simulink model "PerturbedMeanOrbitPropagator"  (R2023a)
settings: Solver=ode4  StartTime=0.0  StopTime=10.0  FixedStep=dt  MaxStep=max_step_size  RelTol=relative_tolerance
undefined symbols (not defined in the file or in its folder): J2_flag, srp_flag
settings Model: Creator=ndelurgio  LastModifiedBy=ndelurgio

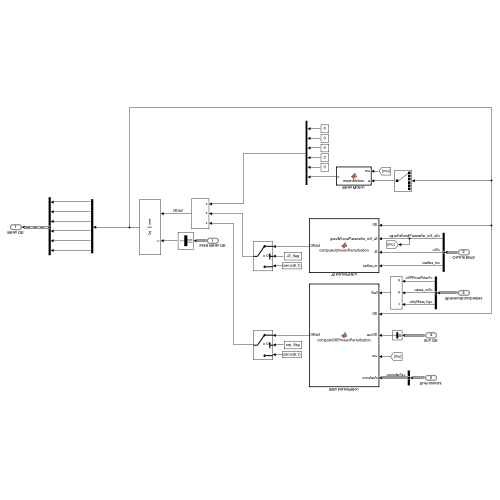
[thumbnail: Simulink's stored preview of the top-level diagram]
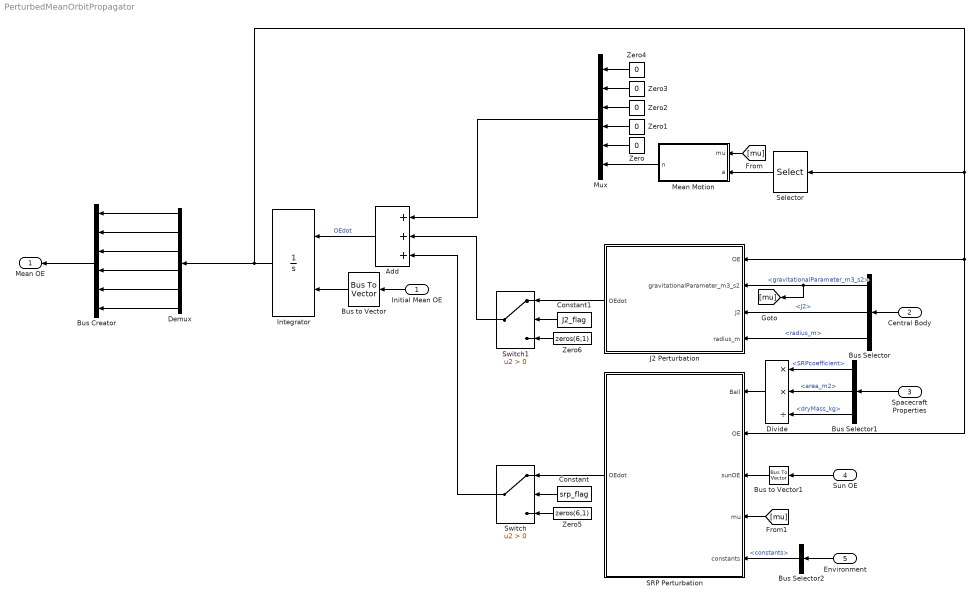
== system PerturbedMeanOrbitPropagator ==
  Initial Mean OE : Inport  OutDataTypeStr=Bus: meanOrbitElements
  Central Body : Inport  Port=2  OutDataTypeStr=Bus: planetProperties
  Spacecraft Properties : Inport  Port=3  OutDataTypeStr=Bus: properties
  Sun OE : Inport  Port=4  OutDataTypeStr=Bus: osculatingOrbitElements
  Environment : Inport  Port=5  OutDataTypeStr=Bus: environmentBus
  Add : Sum  Inputs=+++
  Bus Creator : BusCreator  Inputs=6  OutDataTypeStr=Bus: meanOrbitElements  NonVirtualBus=on
      settings: InheritFromInputs=off
  Bus Selector : BusSelector  OutputSignals=gravitationalParameter_m3_s2,J2,radius_m
  Bus Selector1 : BusSelector  OutputSignals=SRPcoefficient,area_m2,dryMass_kg
  Bus Selector2 : BusSelector  OutputSignals=constants
  Bus to Vector : BusToVector
  Bus to Vector1 : BusToVector
  Constant : Constant  Value=srp_flag
  Constant1 : Constant  Value=J2_flag
  Demux : Demux  Outputs=6
  Divide : Product  Inputs=**/
  Integrator : Integrator  InitialConditionSource=external
  J2 Perturbation : MATLAB Function  TreatAsAtomicUnit=on
  Mean Motion : MATLAB Function  TreatAsAtomicUnit=on
  Mux : Mux  Inputs=6
  SRP Perturbation : MATLAB Function  TreatAsAtomicUnit=on
  Selector : Selector  InputPortWidth=6  IndexOptions=Index vector (dialog)  Indices=[1]  OutputSizes=1
  Switch : Switch  Criteria=u2 > Threshold  SaturateOnIntegerOverflow=off  InputSameDT=off
  Switch1 : Switch  Criteria=u2 > Threshold  SaturateOnIntegerOverflow=off  InputSameDT=off
  Zero{,1..4} (5 alike) : Constant  Value=0  OutDataTypeStr=Inherit: Inherit via back propagation
  Zero5 : Constant  Value=zeros(6,1)  OutDataTypeStr=Inherit: Inherit via back propagation
  Zero6 : Constant  Value=zeros(6,1)  OutDataTypeStr=Inherit: Inherit via back propagation
  Mean OE : Outport  OutDataTypeStr=Bus: meanOrbitElements
  wires:
  Initial Mean OE/1 -> Bus to Vector/1
  Bus to Vector/1 -> Integrator/2
  Add/1 -> Integrator/1  "OEdot"
  Mean Motion/1(n) -> Mux/6
  Zero/1 -> Mux/5
  Zero1/1 -> Mux/4
  Zero2/1 -> Mux/3
  Zero3/1 -> Mux/2
  Zero4/1 -> Mux/1
  Mux/1 -> Add/1
  Integrator/1 -> Demux/1, Selector/1, J2 Perturbation/1(OE), SRP Perturbation/2(OE)
  Selector/1 -> Mean Motion/2(a)
  Central Body/1 -> Bus Selector/1
  Bus Selector/2 -> J2 Perturbation/3(J2)  "<J2>"
  Bus Selector/1 -> [mu], J2 Perturbation/2(gravitationalParameter_m3_s2)  "<gravitationalParameter_m3_s2>"
  Bus Selector/3 -> J2 Perturbation/4(radius_m)  "<radius_m>"
  [mu] -> Mean Motion/1(mu)
  SRP Perturbation/1(OEdot) -> Switch/1
  [mu] -> SRP Perturbation/4(mu)
  Spacecraft Properties/1 -> Bus Selector1/1
  Sun OE/1 -> Bus to Vector1/1
  Bus to Vector1/1 -> SRP Perturbation/3(sunOE)
  Bus Selector1/1 -> Divide/1  "<SRPcoefficient>"
  Bus Selector1/2 -> Divide/2  "<area_m2>"
  Divide/1 -> SRP Perturbation/1(Ball)
  Bus Selector1/3 -> Divide/3  "<dryMass_kg>"
  Bus Selector2/1 -> SRP Perturbation/5(constants)  "<constants>"
  Environment/1 -> Bus Selector2/1
  Demux/1 -> Bus Creator/1
  Demux/2 -> Bus Creator/2
  Demux/3 -> Bus Creator/3
  Demux/4 -> Bus Creator/4
  Demux/5 -> Bus Creator/5
  Demux/6 -> Bus Creator/6
  Bus Creator/1 -> Mean OE/1
  Constant/1 -> Switch/2
  Zero5/1 -> Switch/3
  Switch/1 -> Add/3
  J2 Perturbation/1(OEdot) -> Switch1/1
  Zero6/1 -> Switch1/3
  Constant1/1 -> Switch1/2
  Switch1/1 -> Add/2

== matlab function PerturbedMeanOrbitPropagator/J2 Perturbation ==
  data: OE input; OEdot output; gravitationalParameter_m3_s2 input; J2 input; radius_m input
function OEdot = computeJ2meanPerturbation(OE,gravitationalParameter_m3_s2,J2,radius_m)
OEdot = computeJ2meanPerturbation(OE,gravitationalParameter_m3_s2,J2,radius_m);
end

== matlab function PerturbedMeanOrbitPropagator/Mean Motion ==
  data: mu input; n output; a input
function n = meanMotion (mu, a)
n = meanMotion (mu, a);
end

== matlab function PerturbedMeanOrbitPropagator/SRP Perturbation ==
  data: Ball input; OEdot output; OE input; sunOE input; mu input; constants input
function OEdot = computeSRPmeanPerturbation(Ball, OE, sunOE, mu, constants)
OEdot = computeSRPmeanPerturbation(Ball, OE, sunOE, mu, constants);
end
